simulink model "main_model"  (R2025b)
settings: Solver=FixedStepDiscrete  StartTime=0.0  StopTime=10.0  FixedStep=1e-4  RelTol=1e-3
undefined symbols (not defined in the file or in its folder): dspblkCoreblockFVToolHelper, gcbh
libraries: simulink x6, dspfdesign x1, dspstat3 x1

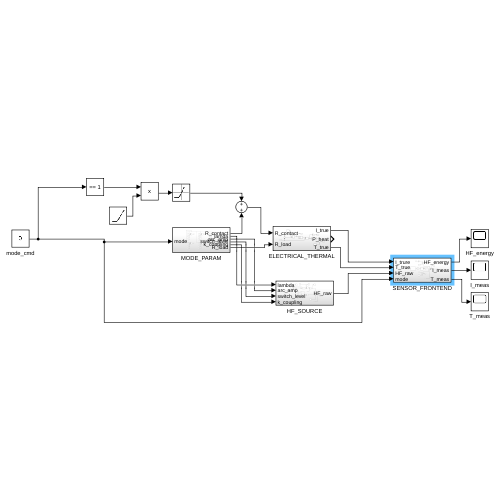
[thumbnail: Simulink's stored preview of the top-level diagram]
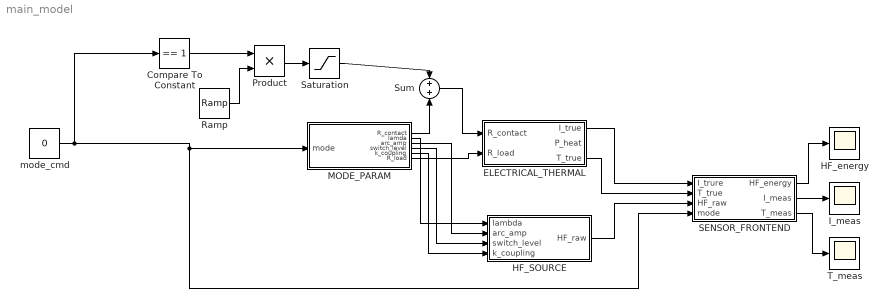
== system main_model ==
  Compare To Constant : simulink/Logic and Bit Operations/Compare To Constant  relop===  const=1  OutDataTypeStr=boolean
  ELECTRICAL_THERMAL : Subsystem
  HF_SOURCE : Subsystem
  HF_energy : Scope
      settings: ActiveDisplayYMinimum=-0.078292607400767572  ActiveDisplayYMaximum=0.70464206405872665
  I_meas : Scope
      settings: ActiveDisplayYMinimum=-209.09631630294618  ActiveDisplayYMaximum=207.20339945692962
  MODE_PARAM : Subsystem
  Product : Product
  Ramp : simulink/Sources/Ramp  slope=0.002  start=0  InitialOutput=0
  SENSOR_FRONTEND : Subsystem
  Saturation : Saturate  UpperLimit=0.05  LowerLimit=0
  Sum : Sum
  T_meas : Scope
      settings: ActiveDisplayYMinimum=-87.513888611775457  ActiveDisplayYMaximum=259.84691774663668  DataLoggingVariableName=ScopeData2
  mode_cmd : Constant  Value=0
  wires:
  MODE_PARAM/2(lamda) -> HF_SOURCE/1(lambda)
  MODE_PARAM/3(arc_amp) -> HF_SOURCE/2(arc_amp)
  MODE_PARAM/4(switch_level) -> HF_SOURCE/3(switch_level)
  MODE_PARAM/5(k_coupling) -> HF_SOURCE/4(k_coupling)
  ELECTRICAL_THERMAL/1(I_true) -> SENSOR_FRONTEND/1(I_trure)
  ELECTRICAL_THERMAL/3(T_true) -> SENSOR_FRONTEND/2(T_true)
  HF_SOURCE/1(HF_raw) -> SENSOR_FRONTEND/3(HF_raw)
  mode_cmd/1 -> SENSOR_FRONTEND/4(mode), MODE_PARAM/1(mode), Compare To Constant/1
  Compare To Constant/1 -> Product/1
  Ramp/1 -> Product/2
  Product/1 -> Saturation/1
  Saturation/1 -> Sum/1
  MODE_PARAM/1(R_contact) -> Sum/2
  Sum/1 -> ELECTRICAL_THERMAL/1(R_contact)
  SENSOR_FRONTEND/2(I_meas) -> I_meas/1
  SENSOR_FRONTEND/3(T_meas) -> T_meas/1
  SENSOR_FRONTEND/1(HF_energy) -> HF_energy/1
  MODE_PARAM/6(R_load) -> ELECTRICAL_THERMAL/2(R_load)

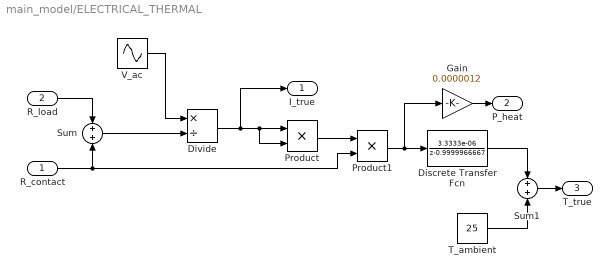
== system main_model/ELECTRICAL_THERMAL ==
  R_contact : Inport
  R_load : Inport  Port=2
  Discrete Transfer Fcn : DiscreteTransferFcn  LoadFcn=dspblkCoreblockFVToolHelper(gcbh,'load');  Numerator=[3.3333e-06]  Denominator=[1 -0.9999966667]
      settings: CopyFcn=dspblkCoreblockFVToolHelper(gcbh,'copy');  DeleteFcn=dspblkCoreblockFVToolHelper(gcbh,'close');  ModelCloseFcn=dspblkCoreblockFVToolHelper(gcbh,'close');  PreSaveFcn=dspblkCoreblockFVToolHelper(gcbh,'presave');  PostSaveFcn=dspblkCoreblockFVToolHelper(gcbh,'postsave');  CloseFcn=dspblkCoreblockFVToolHelper(gcbh,'close');
  Divide : Product  Inputs=*/
  Gain : Gain  Gain=0.0000012
  Product : Product
  Product1 : Product
  Sum : Sum
  Sum1 : Sum
  T_ambient : Constant  Value=25
  V_ac : Sin  Amplitude=1311  Frequency=2*pi*60  SampleTime=1e-4
  I_true : Outport
  P_heat : Outport  Port=2
  T_true : Outport  Port=3
  wires:
  R_load/1 -> Sum/1
  R_contact/1 -> Product1/2, Sum/2
  Sum/1 -> Divide/2
  V_ac/1 -> Divide/1
  Divide/1 -> Product/2, Product/1, I_true/1
  Product/1 -> Product1/1
  Product1/1 -> Gain/1, Discrete Transfer Fcn/1
  Discrete Transfer Fcn/1 -> Sum1/1
  T_ambient/1 -> Sum1/2
  Sum1/1 -> T_true/1
  Gain/1 -> P_heat/1

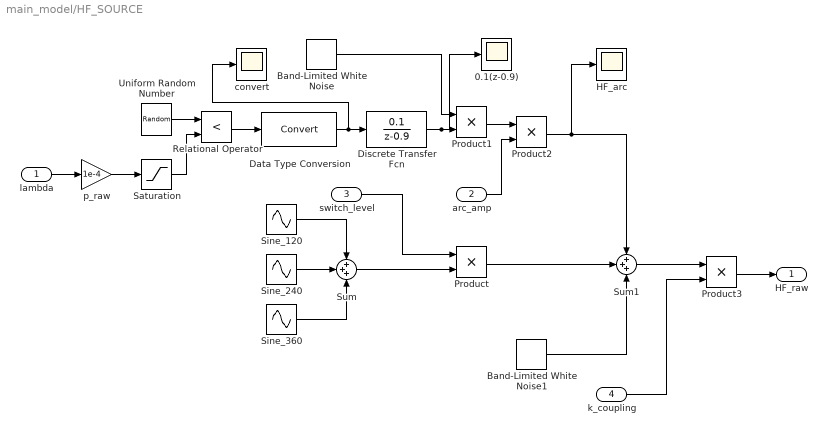
== system main_model/HF_SOURCE ==
  lambda : Inport
  arc_amp : Inport  Port=2
  switch_level : Inport  Port=3
  k_coupling : Inport  Port=4
  0.1(z-0.9) : Scope
      settings: ActiveDisplayYMinimum=-1  ActiveDisplayYMaximum=1  DataLoggingVariableName=ScopeData4
  Band-Limited White Noise : simulink/Sources/Band-Limited White Noise  Cov=1  Ts=1e-4  seed=0
  Band-Limited White Noise1 : simulink/Sources/Band-Limited White Noise  Cov=0.0001  Ts=1e-4  seed=999
  Data Type Conversion : DataTypeConversion  SaturateOnIntegerOverflow=off  RndMeth=Floor
  Discrete Transfer Fcn : DiscreteTransferFcn  LoadFcn=dspblkCoreblockFVToolHelper(gcbh,'load');  Numerator=[0.1]  Denominator=[1 -0.9]
      settings: CopyFcn=dspblkCoreblockFVToolHelper(gcbh,'copy');  DeleteFcn=dspblkCoreblockFVToolHelper(gcbh,'close');  ModelCloseFcn=dspblkCoreblockFVToolHelper(gcbh,'close');  PreSaveFcn=dspblkCoreblockFVToolHelper(gcbh,'presave');  PostSaveFcn=dspblkCoreblockFVToolHelper(gcbh,'postsave');  CloseFcn=dspblkCoreblockFVToolHelper(gcbh,'close');
  HF_arc : Scope
      settings: ActiveDisplayYMinimum=-1  ActiveDisplayYMaximum=1  DataLoggingVariableName=ScopeData5
  Product{,1..3} (4 alike) : Product
  Relational Operator : RelationalOperator  Operator=<  OutDataTypeStr=boolean  RndMeth=Simplest  InputSameDT=off
  Saturation : Saturate  UpperLimit=1  LowerLimit=0
  Sine_120 : Sin  Frequency=2*pi*120  SampleTime=0
  Sine_240 : Sin  Amplitude=0.2  Frequency=2*pi*240  SampleTime=0
  Sine_360 : Sin  Amplitude=0.1  Frequency=2*pi*360  SampleTime=0
  Sum : Sum  Inputs=+++
  Sum1 : Sum  Inputs=+++
  Uniform Random Number : UniformRandomNumber  Minimum=00  SampleTime=1e-4
  convert : Scope
      settings: ActiveDisplayYMinimum=-1  ActiveDisplayYMaximum=1  DataLoggingVariableName=ScopeData3
  p_raw : Gain  Gain=1e-4
  HF_raw : Outport
  wires:
  Sine_240/1 -> Sum/2
  Sine_120/1 -> Sum/1
  Sine_360/1 -> Sum/3
  Sum/1 -> Product/2
  switch_level/1 -> Product/1
  lambda/1 -> p_raw/1
  p_raw/1 -> Saturation/1
  Uniform Random Number/1 -> Relational Operator/1
  Saturation/1 -> Relational Operator/2
  Relational Operator/1 -> Data Type Conversion/1
  arc_amp/1 -> Product2/2
  Product2/1 -> HF_arc/1, Sum1/1
  Product/1 -> Sum1/2
  Band-Limited White Noise1/1 -> Sum1/3
  Sum1/1 -> Product3/1
  k_coupling/1 -> Product3/2
  Product3/1 -> HF_raw/1
  Product1/1 -> Product2/1
  Discrete Transfer Fcn/1 -> 0.1(z-0.9)/1, Product1/2
  Data Type Conversion/1 -> convert/1, Discrete Transfer Fcn/1
  Band-Limited White Noise/1 -> Product1/1

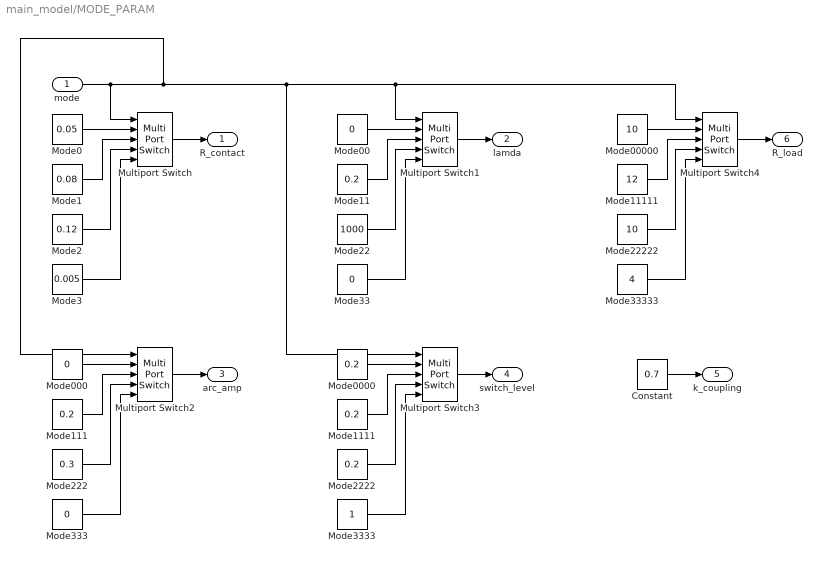
== system main_model/MODE_PARAM ==
  mode : Inport
  Constant : Constant  Value=0.7
  Mode0 : Constant  Value=0.05
  Mode00 : Constant  Value=0
  Mode000 : Constant  Value=0
  Mode0000 : Constant  Value=0.2
  Mode00000 : Constant  Value=10
  Mode1 : Constant  Value=0.08
  Mode{11,111,1111,2222} (4 alike) : Constant  Value=0.2
  Mode11111 : Constant  Value=12
  Mode2 : Constant  Value=0.12
  Mode22 : Constant  Value=1000
  Mode222 : Constant  Value=0.3
  Mode22222 : Constant  Value=10
  Mode3 : Constant  Value=0.005
  Mode33 : Constant  Value=0
  Mode333 : Constant  Value=0
  Mode3333 : Constant
  Mode33333 : Constant  Value=4
  Multiport Switch{,1..4} (5 alike) : MultiPortSwitch  DataPortOrder=Zero-based contiguous  Inputs=4  zeroidx=on  SaturateOnIntegerOverflow=off  InputSameDT=off
  R_contact : Outport
  lamda : Outport  Port=2
  arc_amp : Outport  Port=3
  switch_level : Outport  Port=4
  k_coupling : Outport  Port=5
  R_load : Outport  Port=6
  wires:
  Mode0/1 -> Multiport Switch/2
  Mode1/1 -> Multiport Switch/3
  Mode2/1 -> Multiport Switch/4
  Mode3/1 -> Multiport Switch/5
  mode/1 -> Multiport Switch2/1, Multiport Switch4/1, Multiport Switch1/1, Multiport Switch3/1, Multiport Switch/1
  Multiport Switch/1 -> R_contact/1
  Multiport Switch1/1 -> lamda/1
  Mode33/1 -> Multiport Switch1/5
  Mode22/1 -> Multiport Switch1/4
  Mode11/1 -> Multiport Switch1/3
  Mode00/1 -> Multiport Switch1/2
  Mode000/1 -> Multiport Switch2/2
  Mode111/1 -> Multiport Switch2/3
  Mode222/1 -> Multiport Switch2/4
  Mode333/1 -> Multiport Switch2/5
  Multiport Switch2/1 -> arc_amp/1
  Multiport Switch3/1 -> switch_level/1
  Mode3333/1 -> Multiport Switch3/5
  Mode2222/1 -> Multiport Switch3/4
  Mode1111/1 -> Multiport Switch3/3
  Mode0000/1 -> Multiport Switch3/2
  Constant/1 -> k_coupling/1
  Mode00000/1 -> Multiport Switch4/2
  Mode11111/1 -> Multiport Switch4/3
  Mode22222/1 -> Multiport Switch4/4
  Mode33333/1 -> Multiport Switch4/5
  Multiport Switch4/1 -> R_load/1

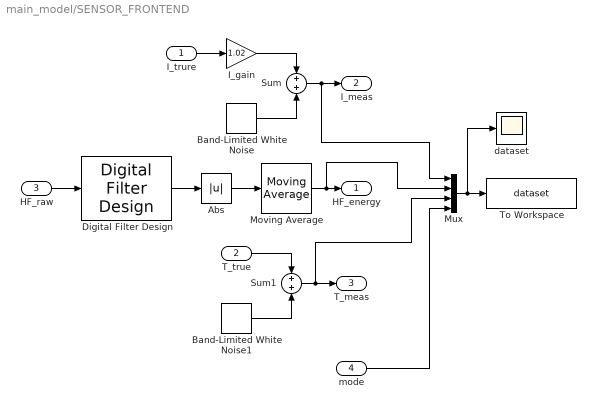
== system main_model/SENSOR_FRONTEND ==
  I_trure : Inport
  T_true : Inport  Port=2
  HF_raw : Inport  Port=3
  mode : Inport  Port=4
  Abs : Abs  SaturateOnIntegerOverflow=off
  Band-Limited White Noise : simulink/Sources/Band-Limited White Noise  Cov=0.01  Ts=1e-4  seed=123
  Band-Limited White Noise1 : simulink/Sources/Band-Limited White Noise  Cov=0.05  Ts=1e-4  seed=456
  Digital Filter Design : dspfdesign/Digital Filter Design  mwdsp_browser_bugfix_var=off
  I_gain : Gain  Gain=1.02
  Moving Average : dspstat3/Moving Average  Method=Sliding window  ForgettingFactorPort=off  SpecifyWindowLength=on  WindowLength=50  OverlapLength=49  AllowArbitraryInputLength=off  ForgettingFactor=0.9  SimulateUsing=Interpreted execution
  Mux : Mux
  Sum : Sum
  Sum1 : Sum
  To Workspace : ToWorkspace  VariableName=dataset  SampleTime=-1
  dataset : Scope
      settings: ActiveDisplayYMinimum=-217.567274506765  ActiveDisplayYMaximum=274.29729395719107  DataLoggingVariableName=ScopeData6
  HF_energy : Outport
  I_meas : Outport  Port=2
  T_meas : Outport  Port=3
  wires:
  Abs/1 -> Moving Average/1
  Moving Average/1 -> Mux/2, HF_energy/1
  I_trure/1 -> I_gain/1
  I_gain/1 -> Sum/1
  Band-Limited White Noise/1 -> Sum/2
  Sum/1 -> Mux/1, I_meas/1
  T_true/1 -> Sum1/1
  Band-Limited White Noise1/1 -> Sum1/2
  Sum1/1 -> Mux/3, T_meas/1
  Mux/1 -> dataset/1, To Workspace/1
  mode/1 -> Mux/4
  HF_raw/1 -> Digital Filter Design/1
  Digital Filter Design/1 -> Abs/1
